simulink model "MSFartoystyringtask14"  (Simulink 8.5)
settings: Solver=ode45  StartTime=tstart  StopTime=tstop  RelTol=1e-3
values from neighbouring files (symbols this model uses):
  amp = 0.3    [run_task_1_4.m]
  c = 1    [run_task_1_4.m]
  K_d = (2*omega_n*T-1)/K    [run_task_1_4.m]
  K_i = omega_n/10*K_p    [run_task_1_4.m]
  K_p = omega_n^2*T/K    [run_task_1_4.m]
  n_c = 7.3    [run_task_1_4.m]
  omega_d = 0.008    [run_task_1_4.m]
  psi0 = 0    [run_task_1_4.m]
  r0 = 0    [run_task_1_4.m]
  tsamp = 10    [run_task_1_4.m]
  v0 = [6.63 0]'    [run_task_1_4.m]
undefined symbols (not defined in the file or in its folder): msfartoystyring
undefined symbols (not defined in the file): p0
settings Model: Creator=christh  LastModifiedBy=ONL  ExtModeAutoUpdateStatusClock=off
settings OptimizationCC: InitFltsAndDblsToZero=on
settings DebuggingCC: SolverPrmCheckMsg=warning  FcnCallInpInsideContextMsg=UseLocalSettings

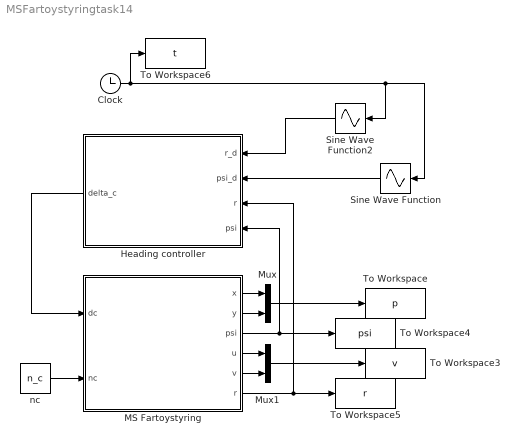
== system MSFartoystyringtask14 ==
  Clock : Clock
  Heading controller : Subsystem
  MS Fartoystyring : Subsystem  mask(MS Fartoystyring for Assignment 3 G&C){x0=p0(1), y0=p0(2), u0=v0(1), v0=v0(2), psi0=psi0, r0=r0, c=c}
      mask prompts: x0 "x(t0) (m)"; y0 "y(t0) (m)"; u0 "u(t0) (m/s)"; v0 "v(t0) (m/s)"; psi0 "psi(t0) (rad)"; r0 "r(t0) (rad/s)"; c "current (0 or 1)"
      mask help:
      | Block corresponding to Figure 1 in the assignment text. Gives the response of the ship.
      |
      | The design speed of MS Fartoystyring is u=8.23 m/s.
      |
      | Input:
      | dc: commanded rudder (rad), dmax=25*pi/180
      | nc: commanded shaft speed (rad/s), nmax=85*2*pi/60
      |
      | Output:
      | x: north pos (m)
      | y: east pos (m)
      | u: surge (m/s)
      | v: sway (m/s)
      | psi: heading (rad)
      | r: yaw (rad/s)
      mask Help: Comments, bugs and help requests can be directed to the TA. Email on course website.
  Mux : Mux  Inputs=2
  Mux1 : Mux  Inputs=2
  Sine Wave Function : Sin  TimeSource=Use external signal  Amplitude=-amp  Frequency=omega_d  SampleTime=0
  Sine Wave Function2 : Sin  TimeSource=Use external signal  Amplitude=-amp*omega_d  Frequency=omega_d  Phase=pi/2  SampleTime=0
  To Workspace : ToWorkspace  VariableName=p  SampleTime=tsamp
  To Workspace3 : ToWorkspace  VariableName=v  SampleTime=tsamp
  To Workspace4 : ToWorkspace  VariableName=psi  SampleTime=tsamp
  To Workspace5 : ToWorkspace  VariableName=r  SampleTime=tsamp
  To Workspace6 : ToWorkspace  VariableName=t  SampleTime=tsamp
  nc : Constant  Value=n_c
  wires:
  Clock/1 -> Sine Wave Function2/1, Sine Wave Function/1, To Workspace6/1
  MS Fartoystyring/1(x) -> Mux/1
  MS Fartoystyring/2(y) -> Mux/2
  MS Fartoystyring/4(u) -> Mux1/1
  MS Fartoystyring/5(v) -> Mux1/2
  Mux/1 -> To Workspace/1
  Mux1/1 -> To Workspace3/1
  MS Fartoystyring/3(psi) -> Heading controller/4(psi), To Workspace4/1
  MS Fartoystyring/6(r) -> Heading controller/3(r), To Workspace5/1
  nc/1 -> MS Fartoystyring/2(nc)
  Heading controller/1(delta_c) -> MS Fartoystyring/1(dc)
  Sine Wave Function/1 -> Heading controller/2("psi_d ")
  Sine Wave Function2/1 -> Heading controller/1("r_d ")

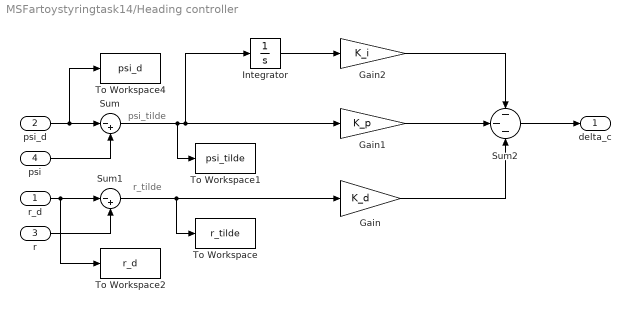
== system MSFartoystyringtask14/Heading controller ==
  note: r_tilde
  note: psi_tilde
  "r_d " : Inport
  "psi_d " : Inport  Port=2
  r : Inport  Port=3
  psi : Inport  Port=4
  Gain : Gain  Gain=K_d
  Gain1 : Gain  Gain=K_p
  Gain2 : Gain  Gain=K_i
  Integrator : Integrator
  Sum : Sum  Inputs=|-+
  Sum1 : Sum  Inputs=|-+
  Sum2 : Sum  Inputs=---
  To Workspace : ToWorkspace  VariableName=r_tilde  SampleTime=tsamp
  To Workspace1 : ToWorkspace  VariableName=psi_tilde  SampleTime=tsamp
  To Workspace2 : ToWorkspace  VariableName=r_d  SampleTime=tsamp
  To Workspace4 : ToWorkspace  VariableName=psi_d  SampleTime=tsamp
  delta_c : Outport
  wires:
  Sum1/1 -> To Workspace/1, Gain/1
  Sum/1 -> To Workspace1/1, Integrator/1, Gain1/1
  Sum2/1 -> delta_c/1
  Gain1/1 -> Sum2/2
  Gain/1 -> Sum2/3
  Gain2/1 -> Sum2/1
  Integrator/1 -> Gain2/1
  "r_d "/1 -> To Workspace2/1, Sum1/1
  r/1 -> Sum1/2
  psi/1 -> Sum/2
  "psi_d "/1 -> To Workspace4/1, Sum/1

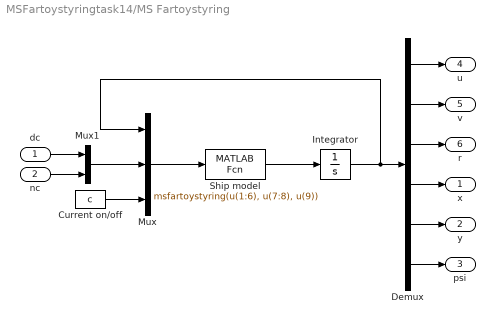
== system MSFartoystyringtask14/MS Fartoystyring ==
  dc : Inport
  nc : Inport  Port=2
  Current on/off : Constant  Value=c
  Demux : Demux  Outputs=6
  Integrator : Integrator  InitialCondition=[u0 v0 r0 x0 y0 psi0]'
  Mux : Mux  Inputs=3
  Mux1 : Mux  Inputs=2
  Ship model : MATLABFcn  MATLABFcn=msfartoystyring(u(1:6), u(7:8), u(9))  OutputDimensions=6
  x : Outport
  y : Outport  Port=2
  psi : Outport  Port=3
  u : Outport  Port=4
  v : Outport  Port=5
  r : Outport  Port=6
  wires:
  Integrator/1 -> Mux/1, Demux/1
  Mux1/1 -> Mux/2
  dc/1 -> Mux1/1
  nc/1 -> Mux1/2
  Demux/1 -> u/1
  Demux/2 -> v/1
  Demux/3 -> r/1
  Demux/4 -> x/1
  Demux/5 -> y/1
  Demux/6 -> psi/1
  Current on/off/1 -> Mux/3
  Ship model/1 -> Integrator/1
  Mux/1 -> Ship model/1
